simulink model "test_Dynamics_EulerPoincare"  (R2021b)
settings: Solver=VariableStepAuto  StartTime=0.0  StopTime=10.0  RelTol=1e-3
InitFcn:
  | % ************** Initiate forces
  | % f0=[0;0;0;0;0;0];
  | % f0=[0;0;0;0;0;0;0];
  | f_0=[0;0;0];
  | f_m=[0;0];
  | f_e=[0;0;0;0;0;0];
  | % ************** Initiate states
  | q_m=[0;0];
  | q_dot_m=[0;0];
  | P=[0;0;0];
  | V_I0=[0;0;0];
  | % ************** Load main
  | %run(Main.m)
values from neighbouring files (symbols this model uses):
  diag_M = diagonalize(M_frak0, M_frak)    [Internal_KUKA_Main.m]    (also in KUKA_Main.m; Main.m)
  iota0 = eye(6,6)    [Internal_KUKA_Main.m]    (also in KUKA_Main.m; Main.m = [1 0 0; 0 1 0;zeros(3,3);0 0 1])
  Xi_m = Xi_m(1:robot.n*6,1:robot.n)    [Internal_KUKA_Main.m]    (also in KUKA_Main.m)
  Xi_m_matrix = zeros(6*n,n)    [Internal_KUKA_Main.m]    (also in KUKA_Main.m; Main.m)
settings Model: Creator=Bmmog  LastModifiedBy=Bmmog
settings SolverCC: AllowMultiTaskInputOutput=on

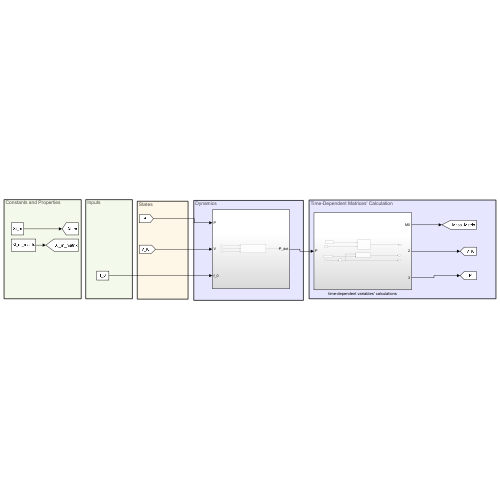
[thumbnail: Simulink's stored preview of the top-level diagram]
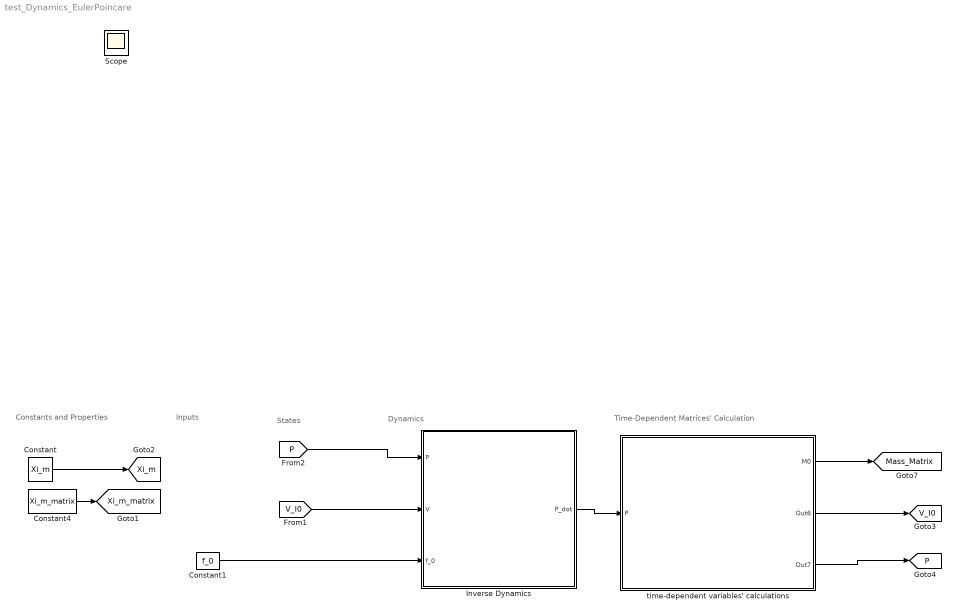
== system test_Dynamics_EulerPoincare ==
  note: Time-Dependent Matrices' Calculation
  note: States
  note: Inputs
  note: Dynamics
  note: Constants and Properties
  Constant : Constant  Value=Xi_m  VectorParams1D=off
  Constant1 : Constant  Value=f_0  VectorParams1D=off
  Constant4 : Constant  Value=Xi_m_matrix  VectorParams1D=off
  Inverse Dynamics : Subsystem
  time-dependent variables' calculations : Subsystem
  Scope : Scope
  tag scope: Mass_Matrix=global, P=global, V_I0=global, Xi_m=global, Xi_m_matrix=global
  wires:
  Constant/1 -> [Xi_m]
  Constant4/1 -> [Xi_m_matrix]
  Constant1/1 -> Inverse Dynamics/3(f_0)
  [P] -> Inverse Dynamics/1(P)
  [V_I0] -> Inverse Dynamics/2(V)
  time-dependent variables' calculations/3(Out7) -> [P]
  time-dependent variables' calculations/2(Out6) -> [V_I0]
  time-dependent variables' calculations/1(M0) -> [Mass_Matrix]
  Inverse Dynamics/1(P_dot) -> time-dependent variables' calculations/1(P)

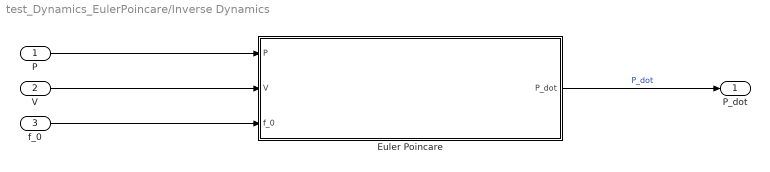
== system test_Dynamics_EulerPoincare/Inverse Dynamics ==
  P : Inport
  V : Inport  Port=2
  f_0 : Inport  Port=3
  Euler Poincare : Subsystem
  P_dot : Outport
  wires:
  f_0/1 -> Euler Poincare/3(f_0)
  Euler Poincare/1(P_dot) -> P_dot/1  "P_dot"
  P/1 -> Euler Poincare/1(P)
  V/1 -> Euler Poincare/2(V)

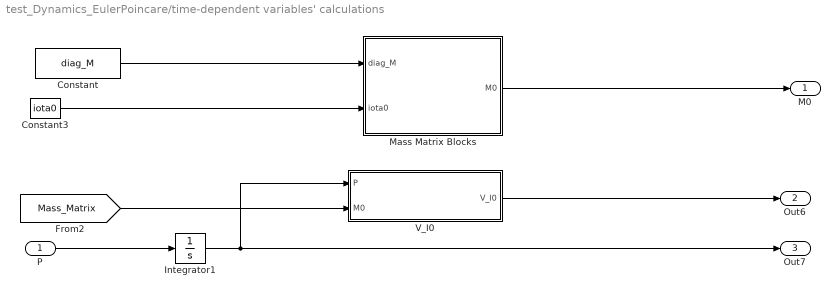
== system test_Dynamics_EulerPoincare/time-dependent variables' calculations ==
  P : Inport
  Constant : Constant  Value=diag_M  VectorParams1D=off
  Constant3 : Constant  Value=iota0  VectorParams1D=off
  Integrator1 : Integrator
  Mass Matrix Blocks : Subsystem
  V_I0 : MATLAB Function  TreatAsAtomicUnit=on
  M0 : Outport
  Out6 : Outport  Port=2
  Out7 : Outport  Port=3
  wires:
  Integrator1/1 -> Out7/1, V_I0/1(P)
  V_I0/1(V_I0) -> Out6/1
  Mass Matrix Blocks/1(M0) -> M0/1
  P/1 -> Integrator1/1
  Constant3/1 -> Mass Matrix Blocks/2(iota0)
  Constant/1 -> Mass Matrix Blocks/1(diag_M)
  [Mass_Matrix] -> V_I0/2(M0)

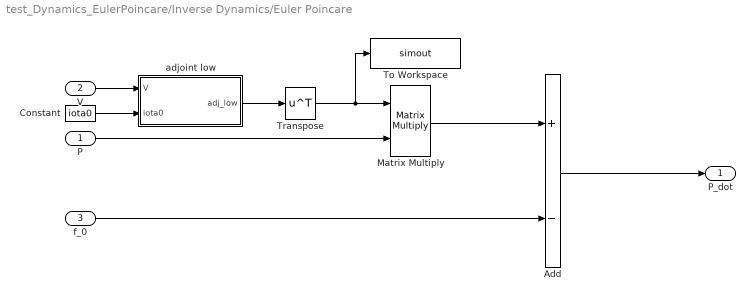
== system test_Dynamics_EulerPoincare/Inverse Dynamics/Euler Poincare ==
  P : Inport
  V : Inport  Port=2
  f_0 : Inport  Port=3
  Add : Sum  Inputs=+-
  Constant : Constant  Value=iota0
  Matrix Multiply : Product  Multiplication=Matrix(*)
  To Workspace : ToWorkspace  VariableName=simout  SaveFormat=Timeseries  SampleTime=-1
  Transpose : Math  Operator=transpose  SaturateOnIntegerOverflow=on
  adjoint low : MATLAB Function  TreatAsAtomicUnit=on
  P_dot : Outport
  wires:
  P/1 -> Matrix Multiply/2
  adjoint low/1(adj_low) -> Transpose/1
  V/1 -> adjoint low/1(V)
  Transpose/1 -> To Workspace/1, Matrix Multiply/1
  Matrix Multiply/1 -> Add/1
  Add/1 -> P_dot/1
  f_0/1 -> Add/2
  Constant/1 -> adjoint low/2(iota0)

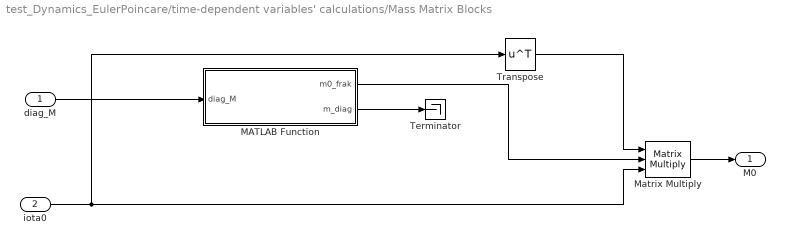
== system test_Dynamics_EulerPoincare/time-dependent variables' calculations/Mass Matrix Blocks ==
  diag_M : Inport
  iota0 : Inport  Port=2
  MATLAB Function : MATLAB Function  TreatAsAtomicUnit=on
  Matrix Multiply : Product  Inputs=3  Multiplication=Matrix(*)
  Terminator : Terminator
  Transpose : Math  Operator=transpose  SaturateOnIntegerOverflow=on
  M0 : Outport
  wires:
  Matrix Multiply/1 -> M0/1
  diag_M/1 -> MATLAB Function/1(diag_M)
  iota0/1 -> Transpose/1, Matrix Multiply/3
  Transpose/1 -> Matrix Multiply/1
  MATLAB Function/2(m_diag) -> Terminator/1
  MATLAB Function/1(m0_frak) -> Matrix Multiply/2

== matlab function test_Dynamics_EulerPoincare/Inverse Dynamics/Euler Poincare/adjoint low ==
  data: V input; adj_low output; iota0 input
function adj_low = adj_low(V, iota0)
% calculates the adjoint corresponding to the Lie bracket of vector V and ()
adj_low = adjoint_low(V,iota0);

== matlab function test_Dynamics_EulerPoincare/time-dependent variables' calculations/Mass Matrix Blocks/MATLAB Function ==
  data: diag_M input; m0_frak output; m_diag output
function [m0_frak,m_diag]=m_frak_decomp(diag_M)
% Compute the Mass Matrix of the multibody system.
%   Output:
%   M0      Spacecraft mass matrix 
%   M0m
%   Mm      Manipulator mass matrix

%n=length(q_m);

m0_frak=diag_M(1:6,1:6);
m_diag=diag_M(7:end,7:end);

== matlab function test_Dynamics_EulerPoincare/time-dependent variables' calculations/V_I0 ==
  data: P input; M0 input; V_I0 output
function V_I0=V_I0(P,M0)
% Find the spaccecraft velocity V_I0
M0_inv=inv(M0);
% temp=P-transpose(A_connection)*q_dot_m;
V_I0=M0_inv\P;
